simulink model "SimuAct6"  (R2025b)
settings: Solver=VariableStepAuto  StartTime=0.0  StopTime=0.005  RelTol=1e-3

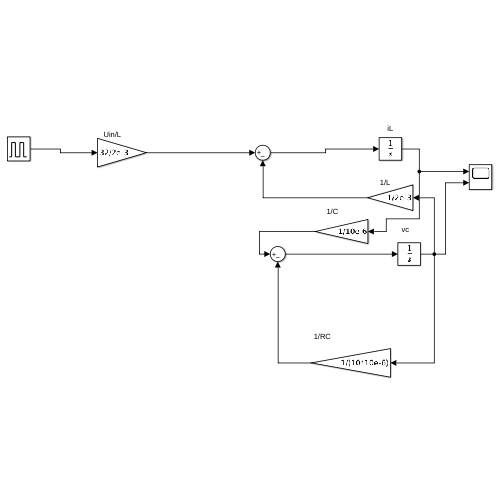
[thumbnail: Simulink's stored preview of the top-level diagram]
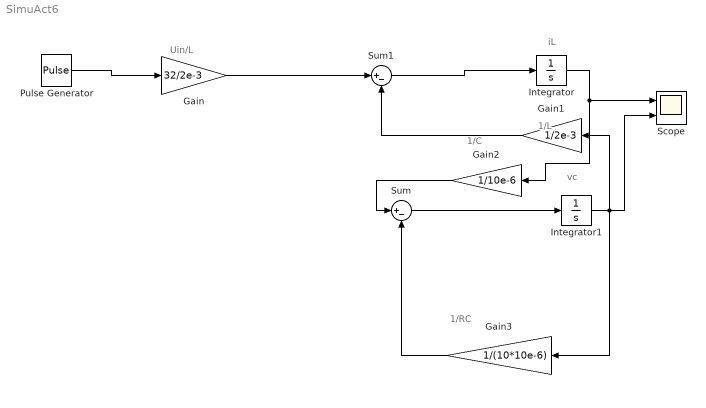
== system SimuAct6 ==
  note: 1/RC
  note: iL
  note: vc
  note: 1/C
  note: 1/L
  note: Uin/L
  Gain : Gain  Gain=32/2e-3
  Gain1 : Gain  Gain=1/2e-3
  Gain2 : Gain  Gain=1/10e-6
  Gain3 : Gain  Gain=1/(10*10e-6)
  Integrator : Integrator
  Integrator1 : Integrator
  Pulse Generator : DiscretePulseGenerator  PulseType=Time based  Period=1/100e3  PulseWidth=40
  Scope : Scope  NumInputPorts=2
      settings: ActiveDisplayYMinimum=-1.6690763206549943  ActiveDisplayYMaximum=15.021686885894953
  Sum : Sum  Inputs=|+-
  Sum1 : Sum  Inputs=|+-
  wires:
  Gain1/1 -> Sum1/2
  Gain/1 -> Sum1/1
  Pulse Generator/1 -> Gain/1
  Sum1/1 -> Integrator/1
  Sum/1 -> Integrator1/1
  Gain2/1 -> Sum/1
  Gain3/1 -> Sum/2
  Integrator/1 -> Gain2/1, Scope/1
  Integrator1/1 -> Gain3/1, Gain1/1, Scope/2
